simulink model "devel"  (R2025a)
settings: Solver=FixedStepAuto  StartTime=0.0  StopTime=15  FixedStep=0.01  MinStep=0.02  RelTol=1e-3
libraries: devel_lib x1
settings Model: Creator=nicolls  LastModifiedBy=nicolls

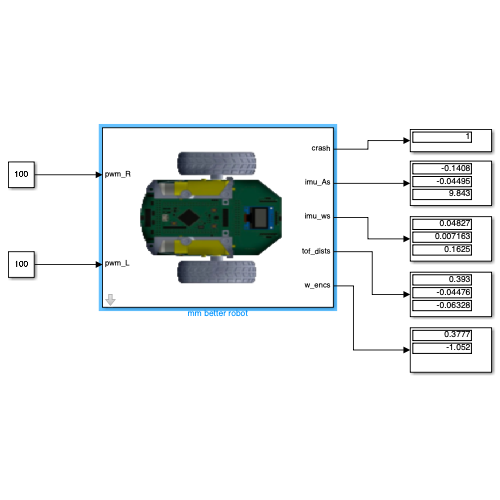
[thumbnail: Simulink's stored preview of the top-level diagram]
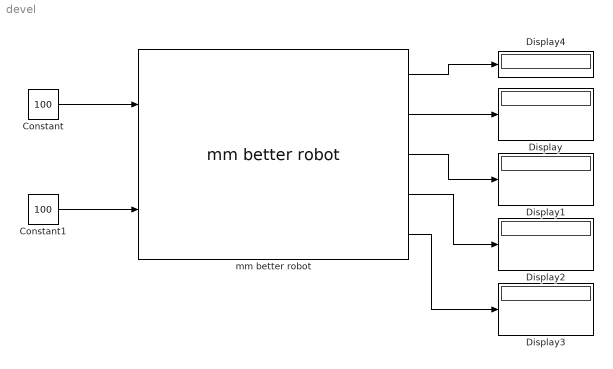
== system devel ==
  Constant : Constant  Value=100
  Constant1 : Constant  Value=100
  Display{,1..4} (5 alike) : Display
  mm better robot : devel_lib/mm better robot  simstruct=simstruct
      link override Random Number5: Variance=0.1^2  Seed=[19 20]
      link override mm simple robot/mm wheel encoders: ticsperrev=8
  wires:
  Constant/1 -> mm better robot/1
  Constant1/1 -> mm better robot/2
  mm better robot/2 -> Display/1
  mm better robot/3 -> Display1/1
  mm better robot/4 -> Display2/1
  mm better robot/5 -> Display3/1
  mm better robot/1 -> Display4/1
